simulink model "RobotModel8"  (R2025b)
settings: Solver=VariableStepAuto  StartTime=0.0  StopTime=150  RelTol=0.01  AbsTol=0.01  EnableMultiTasking=on
values from neighbouring files (symbols this model uses):
  waypoints = [R*cos(theta)+5, R*sin(theta)]    [init_waypoints.m]
undefined symbols (not defined in the file or in its folder): X, Y, Z
libraries: sm_lib x71, nesl_utility x45, slpidlib x2, robotalgslib x1, sharedtransform x1
(part 5 of 5)

== matlab function RobotModel8/FR/MATLAB Function5 ==
  settings: updateMethod=DISCRETE
  data: mode_cmd input; tau output; q input; dq input
function tau = WheelLockPD(mode_cmd, q, dq)
%#codegen
% 针对 Auto 求解器优化的"柔顺刹车"
% 核心思路：滤除噪音 + 限制最大刹车力

% --- 关键参数调整 ---
% 1. 刹车力度上限：大幅降低！
% 前轮是被动轮，很轻，5到10牛米足够锁住了。太大了一定会抖。
tau_max = 10.0;  

% 2. 刹车灵敏度：降低
% 越小越平滑，类似踩刹车时慢慢踩下去，而不是一脚踹死
beta = 5.0;     

% 3. 滤波系数 (0~1)：
% 0.1 表示只有 10% 相信当前的新速度，90% 相信历史速度
% 这能极大地平滑信号，消除仿真震动
filter_alpha = 0.1; 

% --- 状态记忆 ---
persistent dq_smooth
if isempty(dq_smooth), dq_smooth = 0; end

lock = (mode_cmd == 0);

if lock
    % [第一步] 信号滤波 (Low Pass Filter)
    % 这行代码是消除震动的神器
    dq_smooth = (1 - filter_alpha) * dq_smooth + filter_alpha * dq;
    
    % [第二步] 柔和刹车 (Soft Brake)
    % 使用平滑后的速度计算力矩
    friction = tau_max * tanh(beta * dq_smooth);
    
    % 输出反向力矩
    tau = -friction;
    
else
    % 轮式模式：清空滤波器状态，防止切回来时突然跳变
    tau = 0.0;
    dq_smooth = dq; 
end

% 再次限幅（双保险）
if tau > tau_max, tau = tau_max; end
if tau < -tau_max, tau = -tau_max; end

end

== matlab function RobotModel8/RL/MATLAB Function5 ==
  settings: updateMethod=DISCRETE
  data: mode_cmd input; tau output; q input; dq input
function tau = WheelLockPD(mode_cmd, q, dq)
%#codegen
% mode_cmd: 0=Walk (lock wheel), 1=Wheeled (don't lock wheel)
% q, dq measurements from the wheel axle Revolute Joint
% Braking PD parameters (tunable)
Kp = 50.0;     % Braking stiffness, smaller to avoid being too rigid
Kd =  5.0;     % Damping
tau_lim = 150.0;  % Maximum braking torque for the wheel
% Lock only in walk mode
lock = (mode_cmd == 0);
persistent q_hold last_lock
if isempty(q_hold),    q_hold    = q;     end
if isempty(last_lock), last_lock = false; end
% The moment it switches from "unlocked" to "locked", remember the current angle
if (~last_lock) && lock
    q_hold = q;
end
last_lock = lock;
if lock
    % Lock wheel: treat q_hold as the target angle
    q_ref  = q_hold;
    dq_ref = 0.0;
    tau = Kp*(q_ref - q) + Kd*(dq_ref - dq);
else
    % Wheeled mode: do not apply brake
    tau = 0.0;
end
% Torque saturation
if tau >  tau_lim, tau =  tau_lim; end
if tau < -tau_lim, tau = -tau_lim; end
end

== matlab function RobotModel8/RR/MATLAB Function5 ==
  settings: updateMethod=DISCRETE
  data: mode_cmd input; tau output; q input; dq input
function tau = WheelLockPD(mode_cmd, q, dq)
%#codegen
% mode_cmd: 0=Walk (lock wheel), 1=Wheeled (don't lock wheel)
% q, dq measurements from the wheel axle Revolute Joint
% Braking PD parameters (tunable)
Kp = 50.0;     % Braking stiffness, smaller to avoid being too rigid
Kd =  5.0;     % Damping
tau_lim = 150.0;  % Maximum braking torque for the wheel
% Lock only in walk mode
lock = (mode_cmd == 0);
persistent q_hold last_lock
if isempty(q_hold),    q_hold    = q;     end
if isempty(last_lock), last_lock = false; end
% The moment it switches from "unlocked" to "locked", remember the current angle
if (~last_lock) && lock
    q_hold = q;
end
last_lock = lock;
if lock
    % Lock wheel: treat q_hold as the target angle
    q_ref  = q_hold;
    dq_ref = 0.0;
    tau = Kp*(q_ref - q) + Kd*(dq_ref - dq);
else
    % Wheeled mode: do not apply brake
    tau = 0.0;
end
% Torque saturation
if tau >  tau_lim, tau =  tau_lim; end
if tau < -tau_lim, tau = -tau_lim; end
end

== matlab function RobotModel8/FL/MATLAB Function5 ==
  settings: updateMethod=DISCRETE
  data: mode_cmd input; tau output; q input; dq input
function tau = WheelLockPD(mode_cmd, q, dq)
%#codegen
% 针对 Auto 求解器优化的"柔顺刹车"
% 核心思路：滤除噪音 + 限制最大刹车力

% --- 关键参数调整 ---
% 1. 刹车力度上限：大幅降低！
% 前轮是被动轮，很轻，5到10牛米足够锁住了。太大了一定会抖。
tau_max = 10.0;  

% 2. 刹车灵敏度：降低
% 越小越平滑，类似踩刹车时慢慢踩下去，而不是一脚踹死
beta = 5.0;     

% 3. 滤波系数 (0~1)：
% 0.1 表示只有 10% 相信当前的新速度，90% 相信历史速度
% 这能极大地平滑信号，消除仿真震动
filter_alpha = 0.1; 

% --- 状态记忆 ---
persistent dq_smooth
if isempty(dq_smooth), dq_smooth = 0; end

lock = (mode_cmd == 0);

if lock
    % [第一步] 信号滤波 (Low Pass Filter)
    % 这行代码是消除震动的神器
    dq_smooth = (1 - filter_alpha) * dq_smooth + filter_alpha * dq;
    
    % [第二步] 柔和刹车 (Soft Brake)
    % 使用平滑后的速度计算力矩
    friction = tau_max * tanh(beta * dq_smooth);
    
    % 输出反向力矩
    tau = -friction;
    
else
    % 轮式模式：清空滤波器状态，防止切回来时突然跳变
    tau = 0.0;
    dq_smooth = dq; 
end

% 再次限幅（双保险）
if tau > tau_max, tau = tau_max; end
if tau < -tau_max, tau = -tau_max; end

end

== matlab function RobotModel8/FR/MATLAB Function ==
  data: mode_cmd input; alpha input; tau output; q input; dq input; q_cmd input; is_locked output; q_ref output
function [tau, is_locked, q_ref] = LockJointPD(mode_cmd, alpha, q, dq, q_cmd)
%#codegen
% mode_cmd: 0=Walk (track q_cmd), 1=Wheeled (lock current angle)
% alpha   : [0,1] smoothing factor (TransferFcn output), 0=fully walking, 1=fully locked
% q,dq    : joint angle/angular velocity
% q_cmd   : walk/stand target angle (radians)
Kp = 1200.0;   % Starting value, tune per joint
Kd =   20.0;
tau_lim = 300.0;
m = uint8(mode_cmd ~= 0);     % Standardize to uint8(0/1)
a = double(alpha);
persistent q_hold last_mode
if isempty(q_hold),    q_hold    = q;        end   % double
if isempty(last_mode), last_mode = uint8(0); end   % uint8
% Rising edge: 0->1, latch current angle
if (last_mode == uint8(0)) && (m ~= uint8(0))
    q_hold = q;
end
last_mode = m;
% Reference angle: interpolate between "hold angle" and "target angle"
q_ref  = a*q_hold + (1-a)*q_cmd;
dq_ref = 0.0;
% PD
tau = Kp*(q_ref - q) + Kd*(dq_ref - dq);
% Saturation
tau = max(min(tau, tau_lim), -tau_lim);
% Debug flag: is leg lock dominant
is_locked = (a > 0.5);     % Can also output m==1
end

== matlab function RobotModel8/FR/MATLAB Function1 ==
  data: mode_cmd input; alpha input; tau output; q input; dq input; q_cmd input; is_locked output; q_ref output
function [tau, is_locked, q_ref] = LockJointPD(mode_cmd, alpha, q, dq, q_cmd)
%#codegen
% mode_cmd: 0=Walk (track q_cmd), 1=Wheeled (lock current angle)
% alpha   : [0,1] smoothing factor (TransferFcn output), 0=fully walking, 1=fully locked
% q,dq    : joint angle/angular velocity
% q_cmd   : walk/stand target angle (radians)
Kp = 1200.0;   % Starting value, tune per joint
Kd =   20.0;
tau_lim = 300.0;
m = uint8(mode_cmd ~= 0);     % Standardize to uint8(0/1)
a = double(alpha);
persistent q_hold last_mode
if isempty(q_hold),    q_hold    = q;        end   % double
if isempty(last_mode), last_mode = uint8(0); end   % uint8
% Rising edge: 0->1, latch current angle
if (last_mode == uint8(0)) && (m ~= uint8(0))
    q_hold = q;
end
last_mode = m;
% Reference angle: interpolate between "hold angle" and "target angle"
q_ref  = a*q_hold + (1-a)*q_cmd;
dq_ref = 0.0;
% PD
tau = Kp*(q_ref - q) + Kd*(dq_ref - dq);
% Saturation
tau = max(min(tau, tau_lim), -tau_lim);
% Debug flag: is leg lock dominant
is_locked = (a > 0.5);     % Can also output m==1
end

== matlab function RobotModel8/FL/MATLAB Function ==
  data: mode_cmd input; alpha input; tau output; q input; dq input; q_cmd input; is_locked output; q_ref output
function [tau, is_locked, q_ref] = LockJointPD(mode_cmd, alpha, q, dq, q_cmd)
%#codegen
% mode_cmd: 0=Walk (track q_cmd), 1=Wheeled (lock current angle)
% alpha   : [0,1] smoothing factor (TransferFcn output), 0=fully walking, 1=fully locked
% q,dq    : joint angle/angular velocity
% q_cmd   : walk/stand target angle (radians)
Kp = 1200.0;   % Starting value, tune per joint
Kd =   20.0;
tau_lim = 300.0;
m = uint8(mode_cmd ~= 0);     % Standardize to uint8(0/1)
a = double(alpha);
persistent q_hold last_mode
if isempty(q_hold),    q_hold    = q;        end   % double
if isempty(last_mode), last_mode = uint8(0); end   % uint8
% Rising edge: 0->1, latch current angle
if (last_mode == uint8(0)) && (m ~= uint8(0))
    q_hold = q;
end
last_mode = m;
% Reference angle: interpolate between "hold angle" and "target angle"
q_ref  = a*q_hold + (1-a)*q_cmd;
dq_ref = 0.0;
% PD
tau = Kp*(q_ref - q) + Kd*(dq_ref - dq);
% Saturation
tau = max(min(tau, tau_lim), -tau_lim);
% Debug flag: is leg lock dominant
is_locked = (a > 0.5);     % Can also output m==1
end

== matlab function RobotModel8/FL/MATLAB Function1 ==
  data: mode_cmd input; alpha input; tau output; q input; dq input; q_cmd input; is_locked output; q_ref output
function [tau, is_locked, q_ref] = LockJointPD(mode_cmd, alpha, q, dq, q_cmd)
%#codegen
% mode_cmd: 0=Walk (track q_cmd), 1=Wheeled (lock current angle)
% alpha   : [0,1] smoothing factor (TransferFcn output), 0=fully walking, 1=fully locked
% q,dq    : joint angle/angular velocity
% q_cmd   : walk/stand target angle (radians)
Kp = 1200.0;   % Starting value, tune per joint
Kd =   20.0;
tau_lim = 300.0;
m = uint8(mode_cmd ~= 0);     % Standardize to uint8(0/1)
a = double(alpha);
persistent q_hold last_mode
if isempty(q_hold),    q_hold    = q;        end   % double
if isempty(last_mode), last_mode = uint8(0); end   % uint8
% Rising edge: 0->1, latch current angle
if (last_mode == uint8(0)) && (m ~= uint8(0))
    q_hold = q;
end
last_mode = m;
% Reference angle: interpolate between "hold angle" and "target angle"
q_ref  = a*q_hold + (1-a)*q_cmd;
dq_ref = 0.0;
% PD
tau = Kp*(q_ref - q) + Kd*(dq_ref - dq);
% Saturation
tau = max(min(tau, tau_lim), -tau_lim);
% Debug flag: is leg lock dominant
is_locked = (a > 0.5);     % Can also output m==1
end

== matlab function RobotModel8/RL/MATLAB Function ==
  data: mode_cmd input; alpha input; tau output; q input; dq input; q_cmd input; is_locked output; q_ref output
function [tau, is_locked, q_ref] = LockJointPD(mode_cmd, alpha, q, dq, q_cmd)
%#codegen
% mode_cmd: 0=Walk (track q_cmd), 1=Wheeled (lock current angle)
% alpha   : [0,1] smoothing factor (TransferFcn output), 0=fully walking, 1=fully locked
% q,dq    : joint angle/angular velocity
% q_cmd   : walk/stand target angle (radians)
Kp = 1200.0;   % Starting value, tune per joint
Kd =   20.0;
tau_lim = 300.0;
m = uint8(mode_cmd ~= 0);     % Standardize to uint8(0/1)
a = double(alpha);
persistent q_hold last_mode
if isempty(q_hold),    q_hold    = q;        end   % double
if isempty(last_mode), last_mode = uint8(0); end   % uint8
% Rising edge: 0->1, latch current angle
if (last_mode == uint8(0)) && (m ~= uint8(0))
    q_hold = q;
end
last_mode = m;
% Reference angle: interpolate between "hold angle" and "target angle"
q_ref  = a*q_hold + (1-a)*q_cmd;
dq_ref = 0.0;
% PD
tau = Kp*(q_ref - q) + Kd*(dq_ref - dq);
% Saturation
tau = max(min(tau, tau_lim), -tau_lim);
% Debug flag: is leg lock dominant
is_locked = (a > 0.5);     % Can also output m==1
end
